simulink model "Quadcopter_simulation"  (R2023b)
settings: Solver=VariableStepAuto  StartTime=0.0  StopTime=50  RelTol=1e-3
values from neighbouring files (symbols this model uses):
  g = 9.81    [Quadcopter.m]
  Kd_att = 0.4    [Quadcopter.m]
  Kd_pos = 3    [Quadcopter.m]
  Kd_psi = 1.5    [Quadcopter.m]
  Kd_z = 50    [Quadcopter.m]
  Ki_att = 0    [Quadcopter.m]
  Ki_pos = 0.05    [Quadcopter.m]
  Ki_psi = 0.1    [Quadcopter.m]
  Ki_z = 0    [Quadcopter.m]
  Kp_att = 0.03    [Quadcopter.m]
  Kp_pos = 10    [Quadcopter.m]
  Kp_psi = 1    [Quadcopter.m]
  Kp_z = 30    [Quadcopter.m]
  m = 2.355    [Quadcopter.m]
settings Model: Creator=aoqia  LastModifiedBy=chenchen
settings OptimizationCC: ReuseModelBlockBuffer=off

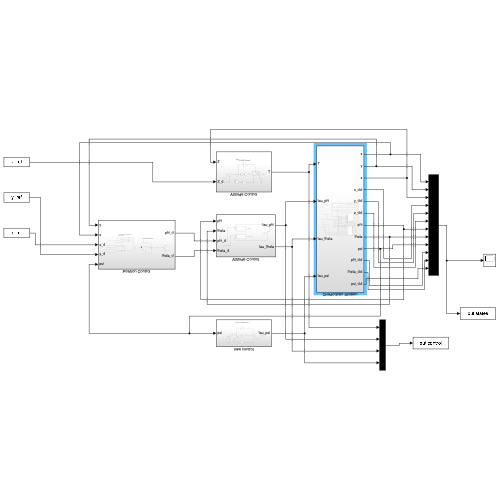
[thumbnail: Simulink's stored preview of the top-level diagram]
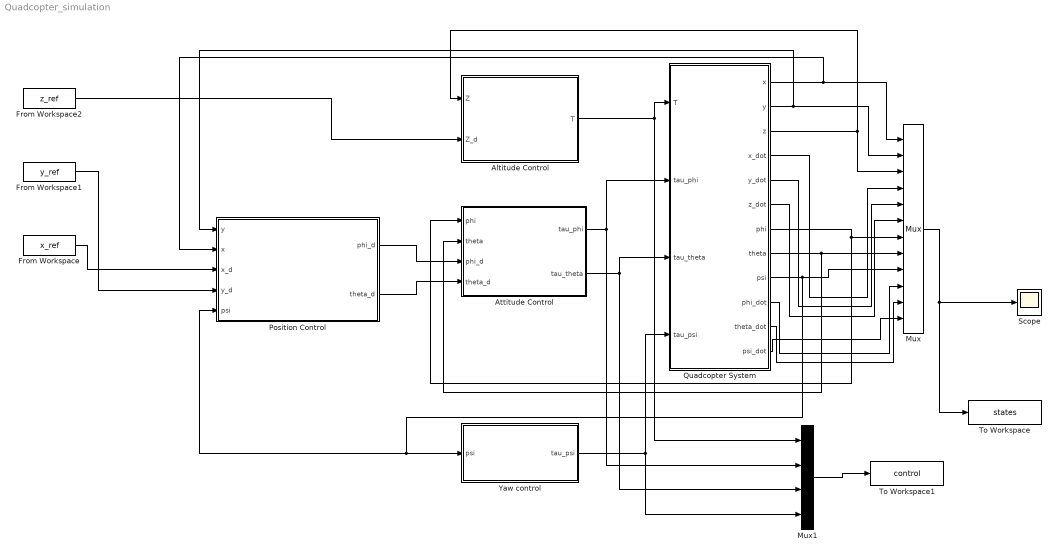
== system Quadcopter_simulation ==
  Altitude Control : Subsystem
  Attitude Control : Subsystem
  From Workspace : FromWorkspace  VariableName=x_ref  OutputAfterFinalValue=Holding final value
  From Workspace1 : FromWorkspace  VariableName=y_ref  OutputAfterFinalValue=Holding final value
  From Workspace2 : FromWorkspace  VariableName=z_ref  OutputAfterFinalValue=Holding final value
  Mux : Mux  Inputs=12
  Mux1 : Mux
  Position Control : Subsystem
  Quadcopter System : Subsystem
  Scope : Scope
  To Workspace : ToWorkspace  VariableName=states  SaveFormat=Timeseries  SampleTime=0.01
  To Workspace1 : ToWorkspace  VariableName=control  SaveFormat=Timeseries  SampleTime=0.01
  Yaw control : Subsystem
  wires:
  Mux/1 -> To Workspace/1, Scope/1
  Quadcopter System/1(x) -> Position Control/2(x), Mux/1
  Quadcopter System/2(y) -> Position Control/1(y), Mux/2
  Quadcopter System/4(x_dot) -> Mux/4
  Quadcopter System/5(y_dot) -> Mux/5
  Quadcopter System/6(z_dot) -> Mux/6
  Quadcopter System/7(phi) -> Attitude Control/1(phi), Mux/7
  Quadcopter System/8(theta) -> Attitude Control/2(theta), Mux/8
  Quadcopter System/9(psi) -> Yaw control/1(psi), Position Control/5(psi), Mux/9
  Quadcopter System/10(phi_dot) -> Mux/10
  Quadcopter System/11(theta_dot) -> Mux/11
  Quadcopter System/12(psi_dot) -> Mux/12
  Altitude Control/1(T) -> Quadcopter System/1(T), Mux1/1
  Quadcopter System/3(z) -> Mux/3, Altitude Control/1(Z)
  From Workspace2/1 -> Altitude Control/2(Z_d)
  Yaw control/1(tau_psi) -> Quadcopter System/4(tau_psi), Mux1/4
  From Workspace1/1 -> Position Control/4(y_d)
  From Workspace/1 -> Position Control/3(x_d)
  Mux1/1 -> To Workspace1/1
  Attitude Control/2(tau_theta) -> Mux1/3, Quadcopter System/3(tau_theta)
  Attitude Control/1(tau_phi) -> Mux1/2, Quadcopter System/2(tau_phi)
  Position Control/1(phi_d) -> Attitude Control/3(phi_d)
  Position Control/2(theta_d) -> Attitude Control/4(theta_d)

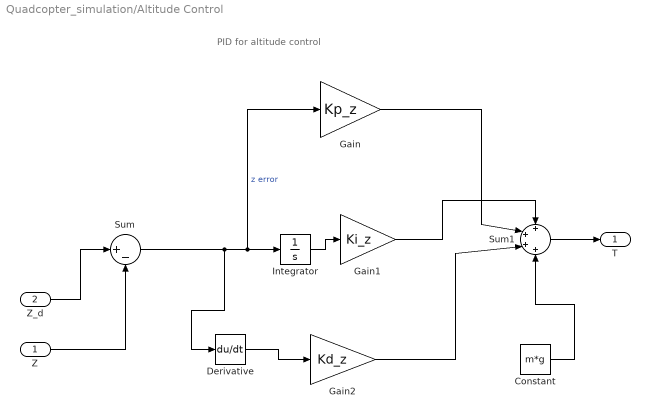
== system Quadcopter_simulation/Altitude Control ==
  note: PID for altitude control
  Z : Inport
  Z_d : Inport  Port=2
  Constant : Constant  Value=m*g
  Derivative : Derivative
  Gain : Gain  Gain=Kp_z
  Gain1 : Gain  Gain=Ki_z
  Gain2 : Gain  Gain=Kd_z
  Integrator : Integrator  LimitOutput=on  UpperSaturationLimit=1  LowerSaturationLimit=-1
  Sum : Sum  Inputs=|+-
  Sum1 : Sum  Inputs=++++
  T : Outport
  wires:
  Z_d/1 -> Sum/1
  Z/1 -> Sum/2
  Derivative/1 -> Gain2/1
  Sum/1 -> Derivative/1, Gain/1, Integrator/1  "z error"
  Gain/1 -> Sum1/2
  Integrator/1 -> Gain1/1
  Sum1/1 -> T/1
  Gain1/1 -> Sum1/1
  Gain2/1 -> Sum1/3
  Constant/1 -> Sum1/4

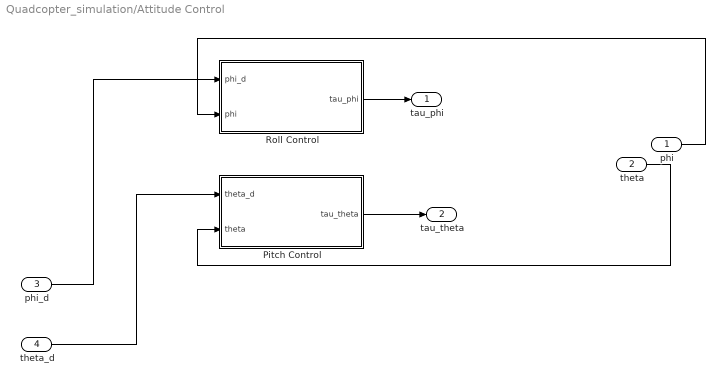
== system Quadcopter_simulation/Attitude Control ==
  phi : Inport
  theta : Inport  Port=2
  phi_d : Inport  Port=3
  theta_d : Inport  Port=4
  Pitch Control : Subsystem
  Roll Control : Subsystem
  tau_phi : Outport
  tau_theta : Outport  Port=2
  wires:
  phi/1 -> Roll Control/2(phi)
  phi_d/1 -> Roll Control/1(phi_d)
  Pitch Control/1(tau_theta) -> tau_theta/1
  theta_d/1 -> Pitch Control/1(theta_d)
  theta/1 -> Pitch Control/2(theta)
  Roll Control/1(tau_phi) -> tau_phi/1

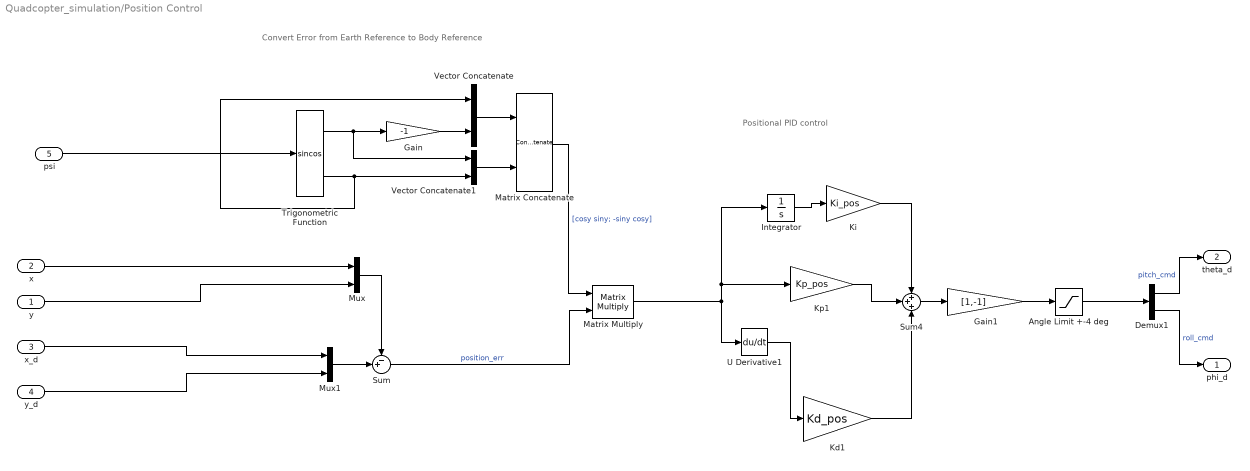
== system Quadcopter_simulation/Position Control ==
  note: Convert Error from Earth Reference to Body Reference
  note: Positional PID control
  y : Inport
  x : Inport  Port=2
  x_d : Inport  Port=3
  y_d : Inport  Port=4
  psi : Inport  Port=5
  Angle Limit +-4 deg : Saturate  UpperLimit=4*pi/180  LowerLimit=-4*pi/180  ZeroCross=off
  Demux1 : Demux  Outputs=2
  Gain : Gain  Gain=-1
  Gain1 : Gain  Gain=[1,-1]
  Integrator : Integrator  LimitOutput=on  UpperSaturationLimit=1  LowerSaturationLimit=-1
  Kd1 : Gain  Gain=Kd_pos
  Ki : Gain  Gain=Ki_pos
  Kp1 : Gain  Gain=Kp_pos
  Matrix Concatenate : Concatenate  Mode=Multidimensional array  ConcatenateDimension=2
  Matrix Multiply : Product  Multiplication=Matrix(*)
  Mux : Mux  Inputs=2
  Mux1 : Mux  Inputs=2
  Sum : Sum  Inputs=-+|
  Sum4 : Sum  Inputs=+++
  Trigonometric Function : Trigonometry  Operator=sincos
  U Derivative1 : Derivative
  Vector Concatenate : Concatenate
  Vector Concatenate1 : Concatenate
  phi_d : Outport
  theta_d : Outport  Port=2
  wires:
  Vector Concatenate1/1 -> Matrix Concatenate/2
  Ki/1 -> Sum4/1
  Kp1/1 -> Sum4/2
  Integrator/1 -> Ki/1
  Matrix Multiply/1 -> Integrator/1, Kp1/1, U Derivative1/1
  U Derivative1/1 -> Kd1/1
  Angle Limit +-4 deg/1 -> Demux1/1
  Trigonometric Function/1 -> Vector Concatenate1/1, Gain/1
  Sum/1 -> Matrix Multiply/2  "position_err"
  x/1 -> Mux/1
  Kd1/1 -> Sum4/3
  psi/1 -> Trigonometric Function/1
  Gain1/1 -> Angle Limit +-4 deg/1
  Matrix Concatenate/1 -> Matrix Multiply/1  "[cosy siny; -siny cosy]"
  Trigonometric Function/2 -> Vector Concatenate1/2, Vector Concatenate/1
  Vector Concatenate/1 -> Matrix Concatenate/1
  Gain/1 -> Vector Concatenate/2
  Sum4/1 -> Gain1/1
  Mux1/1 -> Sum/2
  Mux/1 -> Sum/1
  y/1 -> Mux/2
  x_d/1 -> Mux1/1
  y_d/1 -> Mux1/2
  Demux1/1 -> theta_d/1  "pitch_cmd"
  Demux1/2 -> phi_d/1  "roll_cmd"

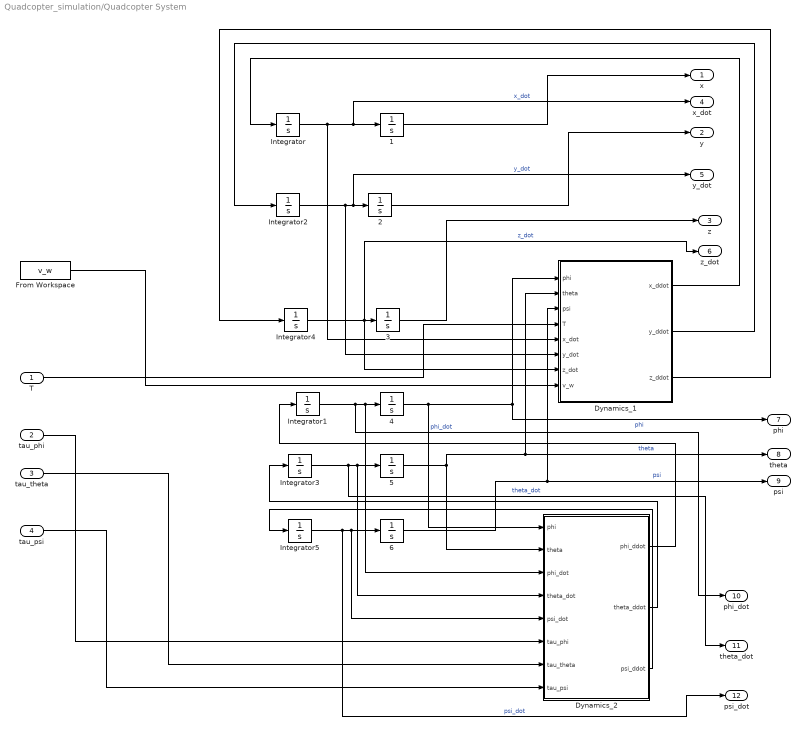
== system Quadcopter_simulation/Quadcopter System ==
  T : Inport
  tau_phi : Inport  Port=2
  tau_theta : Inport  Port=3
  tau_psi : Inport  Port=4
  1 : Integrator
  2 : Integrator
  3 : Integrator  LimitOutput=on  LowerSaturationLimit=0
  4 : Integrator  LimitOutput=on  UpperSaturationLimit=0.34  LowerSaturationLimit=-0.34
  5 : Integrator  LimitOutput=on  UpperSaturationLimit=0.34  LowerSaturationLimit=-0.34
  6 : Integrator  UpperSaturationLimit=pi  LowerSaturationLimit=-pi  WrapState=on  ZeroCross=off
  Dynamics_1 : MATLAB Function  TreatAsAtomicUnit=on
  Dynamics_2 : MATLAB Function  TreatAsAtomicUnit=on
  From Workspace : FromWorkspace  VariableName=v_w
  Integrator{,1..5} (6 alike) : Integrator
  x : Outport
  y : Outport  Port=2
  z : Outport  Port=3
  x_dot : Outport  Port=4
  y_dot : Outport  Port=5
  z_dot : Outport  Port=6
  phi : Outport  Port=7
  theta : Outport  Port=8
  psi : Outport  Port=9
  phi_dot : Outport  Port=10
  theta_dot : Outport  Port=11
  psi_dot : Outport  Port=12
  wires:
  5/1 -> Dynamics_2/2(theta), Dynamics_1/2(theta), theta/1  "theta"
  Integrator/1 -> x_dot/1, 1/1, Dynamics_1/5(x_dot)  "x_dot"
  Integrator2/1 -> Dynamics_1/6(y_dot), y_dot/1, 2/1  "y_dot"
  4/1 -> Dynamics_2/1(phi), Dynamics_1/1(phi), phi/1  "phi"
  Integrator4/1 -> Dynamics_1/7(z_dot), z_dot/1, 3/1  "z_dot"
  Integrator1/1 -> phi_dot/1, Dynamics_2/3(phi_dot), 4/1  "phi_dot"
  Integrator5/1 -> psi_dot/1, Dynamics_2/5(psi_dot), 6/1  "psi_dot"
  Integrator3/1 -> theta_dot/1, Dynamics_2/4(theta_dot), 5/1  "theta_dot"
  1/1 -> x/1
  Dynamics_2/2(theta_ddot) -> Integrator3/1
  tau_theta/1 -> Dynamics_2/7(tau_theta)
  6/1 -> Dynamics_1/3(psi), psi/1  "psi"
  2/1 -> y/1
  tau_psi/1 -> Dynamics_2/8(tau_psi)
  Dynamics_2/1(phi_ddot) -> Integrator1/1
  3/1 -> z/1
  T/1 -> Dynamics_1/4(T)
  Dynamics_2/3(psi_ddot) -> Integrator5/1
  tau_phi/1 -> Dynamics_2/6(tau_phi)
  Dynamics_1/3(z_ddot) -> Integrator4/1
  Dynamics_1/1(x_ddot) -> Integrator/1
  Dynamics_1/2(y_ddot) -> Integrator2/1
  From Workspace/1 -> Dynamics_1/8(v_w)

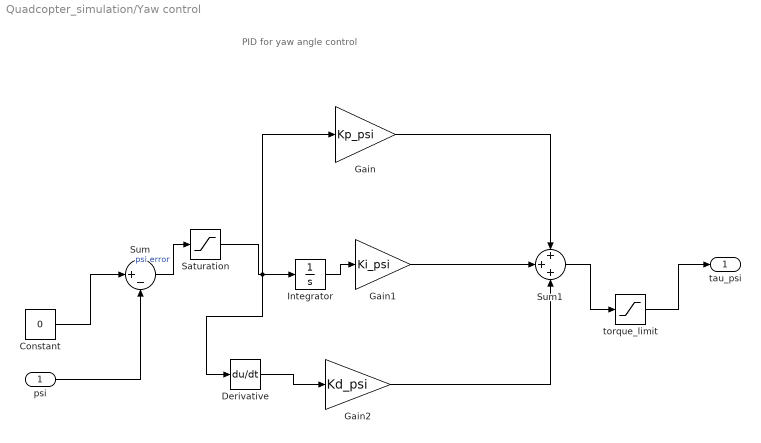
== system Quadcopter_simulation/Yaw control ==
  note: PID for yaw angle control
  psi : Inport
  Constant : Constant  Value=0
  Derivative : Derivative
  Gain : Gain  Gain=Kp_psi
  Gain1 : Gain  Gain=Ki_psi
  Gain2 : Gain  Gain=Kd_psi
  Integrator : Integrator  LimitOutput=on  UpperSaturationLimit=1  LowerSaturationLimit=-1
  Saturation : Saturate  UpperLimit=pi  LowerLimit=-pi
  Sum : Sum  Inputs=|+-
  Sum1 : Sum  Inputs=+++
  torque_limit : Saturate  UpperLimit=5  LowerLimit=-5  ZeroCross=off
  tau_psi : Outport
  wires:
  Constant/1 -> Sum/1
  psi/1 -> Sum/2
  Derivative/1 -> Gain2/1
  Gain/1 -> Sum1/1
  Integrator/1 -> Gain1/1
  Gain1/1 -> Sum1/2
  Gain2/1 -> Sum1/3
  Sum1/1 -> torque_limit/1
  torque_limit/1 -> tau_psi/1
  Sum/1 -> Saturation/1  "psi error"
  Saturation/1 -> Gain/1, Derivative/1, Integrator/1

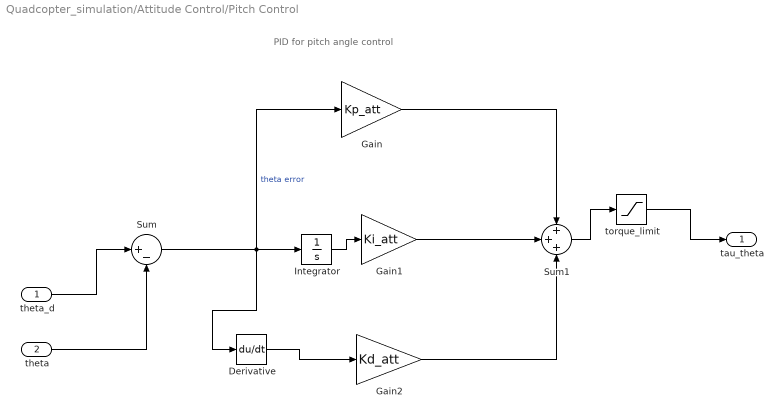
== system Quadcopter_simulation/Attitude Control/Pitch Control ==
  note: PID for pitch angle control
  theta_d : Inport
  theta : Inport  Port=2
  Derivative : Derivative
  Gain : Gain  Gain=Kp_att
  Gain1 : Gain  Gain=Ki_att
  Gain2 : Gain  Gain=Kd_att
  Integrator : Integrator  LimitOutput=on  UpperSaturationLimit=1  LowerSaturationLimit=-1
  Sum : Sum  Inputs=|+-
  Sum1 : Sum  Inputs=+++
  torque_limit : Saturate  UpperLimit=5  LowerLimit=-5  ZeroCross=off
  tau_theta : Outport
  wires:
  theta_d/1 -> Sum/1
  Integrator/1 -> Gain1/1
  Gain1/1 -> Sum1/2
  Sum1/1 -> torque_limit/1
  theta/1 -> Sum/2
  Gain/1 -> Sum1/1
  Sum/1 -> Integrator/1, Gain/1, Derivative/1  "theta error"
  Derivative/1 -> Gain2/1
  Gain2/1 -> Sum1/3
  torque_limit/1 -> tau_theta/1

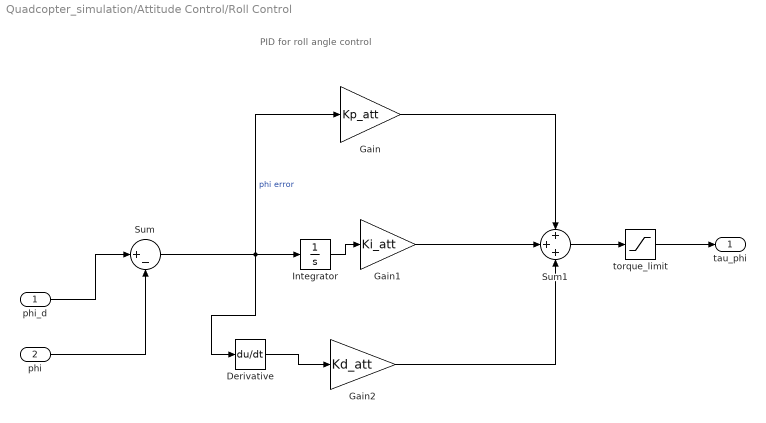
== system Quadcopter_simulation/Attitude Control/Roll Control ==
  note: PID for roll angle control
  phi_d : Inport
  phi : Inport  Port=2
  Derivative : Derivative
  Gain : Gain  Gain=Kp_att
  Gain1 : Gain  Gain=Ki_att
  Gain2 : Gain  Gain=Kd_att
  Integrator : Integrator  LimitOutput=on  UpperSaturationLimit=1  LowerSaturationLimit=-1
  Sum : Sum  Inputs=|+-
  Sum1 : Sum  Inputs=+++
  torque_limit : Saturate  UpperLimit=5  LowerLimit=-5  ZeroCross=off
  tau_phi : Outport
  wires:
  phi_d/1 -> Sum/1
  Integrator/1 -> Gain1/1
  Gain1/1 -> Sum1/2
  Sum1/1 -> torque_limit/1
  phi/1 -> Sum/2
  Gain/1 -> Sum1/1
  Sum/1 -> Integrator/1, Gain/1, Derivative/1  "phi error"
  Derivative/1 -> Gain2/1
  Gain2/1 -> Sum1/3
  torque_limit/1 -> tau_phi/1

== matlab function Quadcopter_simulation/Quadcopter System/Dynamics_2 ==
  data: phi input; phi_ddot output; theta input; phi_dot input; theta_dot input; psi_dot input; tau_phi input; tau_theta input; tau_psi input; theta_ddot output; psi_ddot output
function [phi_ddot, theta_ddot, psi_ddot] = fcn(phi,theta,phi_dot,theta_dot,psi_dot,tau_phi,tau_theta,tau_psi)
Ixx = 4.856*10^-3;
Iyy = 4.856*10^-3;
Izz = 8.801*10^-3;

%%%TODO_3%%%
%Calculate the coriolis matrix
c11 = 0;
c12 = (Iyy-Izz)*(theta_dot*cos(phi)*sin(phi) + psi_dot*cos(theta)*(sin(phi)^2-cos(phi)^2)) - Ixx*psi_dot*cos(theta);
c13 = (Izz-Iyy)*psi_dot*cos(phi)*sin(phi)*cos(theta)^2;
c21 = (Izz-Iyy)*(theta_dot*cos(phi)*sin(phi) + psi_dot*cos(theta)*(sin(phi)^2-cos(phi)^2)) + Ixx*psi_dot*cos(theta);
c22 = (Izz-Iyy)*phi_dot*cos(phi)*sin(phi);
c23 = (-Ixx*psi_dot + Iyy*psi_dot*sin(phi)^2 + Izz*psi_dot*cos(phi)^2)*sin(theta)*cos(theta);
c31 = (Iyy-Izz)*psi_dot*cos(theta)^2*sin(phi)*cos(phi) - Ixx*theta_dot*cos(theta);
c32 = (Izz-Iyy)*(theta_dot*cos(phi)*sin(phi)*sin(theta)+phi_dot*cos(theta)*(sin(phi)^2-cos(phi)^2)) + (Ixx-Iyy*sin(phi)^2-Izz*cos(phi)^2)*psi_dot*sin(theta)*cos(theta);
c33 = (Iyy-Izz)*phi_dot*cos(phi)*sin(phi)*cos(theta)^2 + (Ixx - Iyy*sin(phi)^2 - Izz*cos(phi)^2)*theta_dot*cos(theta)*sin(theta);

C = [c11 c12 c13; c21 c22 c23; c31 c32 c33];


%%%%%%

n_dot = [phi_dot;theta_dot;psi_dot];
tau = [tau_phi;tau_theta;tau_psi];

%%%TODO_4%%%
%Calculate the acceleration
term = tau - (C*n_dot);
W = [1 0 -sin(theta); 0 cos(phi) cos(theta)*sin(phi); 0 -sin(phi) cos(theta)*cos(phi)];
I_B = [Ixx 0 0; 0 Iyy 0; 0 0 Izz];
J = transpose(W)* I_B * W;

output = inv(J)*term;
phi_ddot = output(1);
theta_ddot = output(2);
psi_ddot = output(3);

== matlab function Quadcopter_simulation/Quadcopter System/Dynamics_1 ==
  data: phi input; x_ddot output; theta input; psi input; T input; y_ddot output; z_ddot output; x_dot input; y_dot input; z_dot input; v_w input
function [x_ddot,y_ddot,z_ddot] = fcn(phi,theta,psi,T,x_dot,y_dot,z_dot, v_w)


Ax = 0.25; %Drag coefficient
Ay = 0.25;
Az = 0.25;
g = 9.81;
m = 2.355; %mass of quadcopter

%%%%%TODO_1%%%%%%

%Calculate the rotational matrix R_GB and R_BG

R_GB = [cos(phi)*cos(psi) sin(psi)*cos(phi) -sin(theta);
        cos(psi)*sin(theta)*sin(phi)-sin(psi)*cos(phi) sin(psi)*sin(theta)*sin(phi)+cos(phi)*cos(psi) cos(theta)*sin(phi);
        cos(psi)*sin(theta)*cos(phi)+sin(phi)*sin(psi) sin(psi)*sin(theta)*cos(phi)-cos(psi)*sin(phi) cos(phi)*cos(theta)];

R_BG = transpose(R_GB); %Rotation matrix from body frame to global frame

%Calculate the damping matrix
D = [Ax 0 0;
     0 Ay 0;
     0 0 Az];

rho_air = 1.225; % air density in [kg/m^3]
area = [0.03; 0.03; 0.0848]; % area in m^2
drag_coefficient = 0.9;

%%%%%%TODO_2%%%%%%%%%%%
%Calculate the acceleration

relative_w_dot = R_GB * [v_w(1) - x_dot; v_w(2) - y_dot; v_w(3) - z_dot];

w_ddot = R_BG * 0.5*rho_air * drag_coefficient * (area.* (relative_w_dot.^2) ) / m;
% fprintf("wddot %f, %f, %f\n", w_ddot(1), w_ddot(2), w_ddot(3));

p_ddot = [0;0;-g] + (1/m)*R_BG*[0;0;T] + w_ddot;

% fprintf("wind_ddot x: %f, y:%f, z:%f\n", relative_w_dot(1), relative_w_dot(2), relative_w_dot(3));
% p_ddot = [0;0;-g] + (1/m)*R_BG*[0;0;T] - (1/m)*D*[x_dot;y_dot;z_dot];

x_ddot = p_ddot(1);
y_ddot = p_ddot(2);
z_ddot = p_ddot(3);

% fprintf("pddot %f, %f, %f\n", x_ddot, y_ddot, z_ddot);
